simulink model "EngTemplate_r2017a"  (R2017a)
settings: Solver=ode5  StartTime=0.0  StopTime=inf  FixedStep=0.0001  RelTol=1e-3  EnableMultiTasking=on
values from neighbouring files (symbols this model uses):
  Patm = 101.3e3    (= 101300)    [EngineParameters.m]
settings Model: Creator=bamason2  LastModifiedBy=byronmason
settings DataIOCC: LimitDataPoints=on  SaveFormat=Array
settings OptimizationCC: LifeSpan=inf
settings DebuggingCC: SFUnexpectedBacktrackingDiag=warning  SFNoUnconditionalDefaultTransitionDiag=warning  SFExecutionAtInitializationDiag=none
settings HardwareCC: ProdBitPerPointer=32  ProdBitPerSizeT=32  ProdBitPerPtrDiffT=32  ProdLargestAtomicFloat=None  ProdIntDivRoundTo=Undefined  ProdEndianess=Unspecified  ProdWordSize=32  ProdHWDeviceType=32-bit Generic
settings ModelReferenceCC: PropagateSignalLabelsOutOfModel=off
settings GRTTargetCC: TargetLangStandard=C89/C90 (ANSI)
settings ConfigComp: CovMetricSettings=dw  CovSaveCumulativeToWorkspaceVar=on  CovSaveSingleToWorkspaceVar=on  CovExternalEMLEnable=off

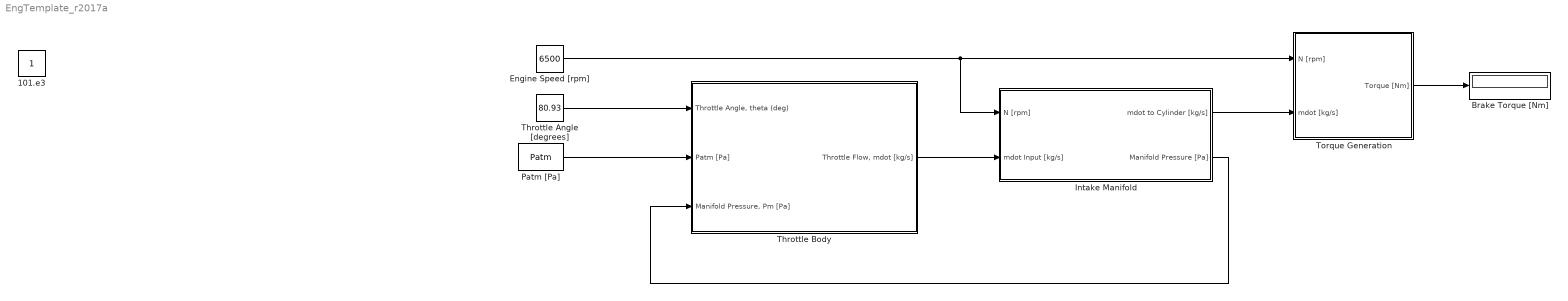
== system EngTemplate_r2017a ==
  Brake Torque [Nm] : Display
  Engine Speed [rpm] : Constant  Value=6500
  Intake Manifold : Subsystem
  Patm [Pa] : Constant  Value=Patm
  Throttle Angle [degrees] : Constant  Value=80.93
  Throttle Body : Subsystem
  Torque Generation : Subsystem
  101.e3 : Constant  IOType=siggen
  wires:
  Intake Manifold/1(mdot to Cylinder [kg/s]) -> Torque Generation/2(mdot [kg/s])
  Torque Generation/1(Torque [Nm]) -> Brake Torque [Nm]/1
  Intake Manifold/2(Manifold Pressure [Pa]) -> Throttle Body/3("Manifold Pressure, Pm [Pa]")
  Throttle Body/1("Throttle Flow, mdot [kg/s]") -> Intake Manifold/2(mdot Input [kg/s])
  Engine Speed [rpm]/1 -> Intake Manifold/1(N [rpm]), Torque Generation/1(N [rpm])
  Throttle Angle [degrees]/1 -> Throttle Body/1("Throttle Angle, theta (deg)")
  Patm [Pa]/1 -> Throttle Body/2(Patm [Pa])

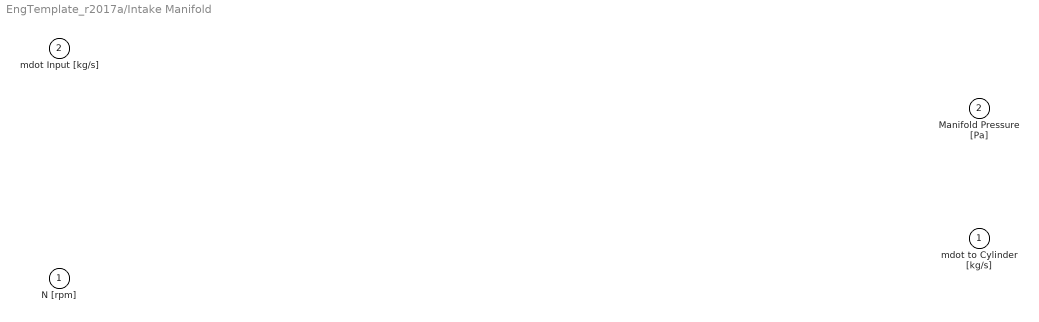
== system EngTemplate_r2017a/Intake Manifold ==
  N [rpm] : Inport
  mdot Input [kg/s] : Inport  Port=2
  mdot to Cylinder [kg/s] : Outport  InitialOutput=0
  Manifold Pressure [Pa] : Outport  Port=2  InitialOutput=0

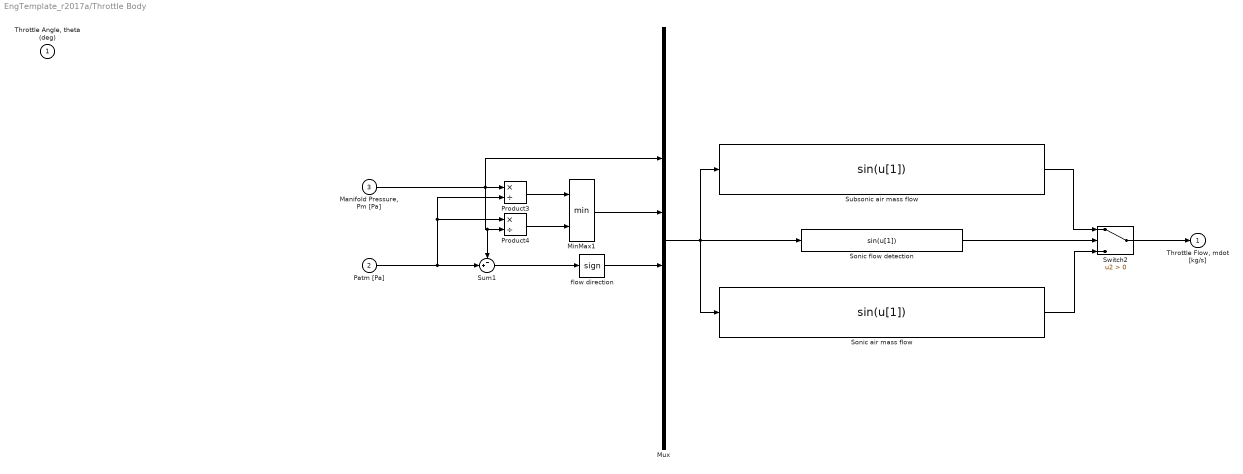
== system EngTemplate_r2017a/Throttle Body ==
  "Throttle Angle, theta (deg)" : Inport
  Patm [Pa] : Inport  Port=2
  "Manifold Pressure, Pm [Pa]" : Inport  Port=3
  MinMax1 : MinMax  Inputs=2  InputSameDT=on  SaturateOnIntegerOverflow=on
  Mux : Mux  Inputs=8
  Product3 : Product  Inputs=*/  InputSameDT=on  RndMeth=Zero  SaturateOnIntegerOverflow=on  OutDataTypeStr=Inherit: Same as first input
  Product4 : Product  Inputs=*/  InputSameDT=on  RndMeth=Zero  SaturateOnIntegerOverflow=on  OutDataTypeStr=Inherit: Same as first input
  Sonic air mass flow : Fcn
  Sonic flow detection : Fcn
  Subsonic air mass flow : Fcn
  Sum1 : Sum  Inputs=-+|  InputSameDT=on  SaturateOnIntegerOverflow=on  OutDataTypeStr=Inherit: Same as first input
  Switch2 : Switch  Criteria=u2 > Threshold
  flow direction : Signum
  "Throttle Flow, mdot [kg/s]" : Outport  InitialOutput=0
  wires:
  Mux/1 -> Sonic air mass flow/1, Subsonic air mass flow/1, Sonic flow detection/1
  Sonic flow detection/1 -> Switch2/2
  Switch2/1 -> "Throttle Flow, mdot [kg/s]"/1
  Subsonic air mass flow/1 -> Switch2/1
  Sonic air mass flow/1 -> Switch2/3
  "Manifold Pressure, Pm [Pa]"/1 -> Product4/2, Sum1/1, Mux/3, Product3/1
  flow direction/1 -> Mux/5
  Patm [Pa]/1 -> Product4/1, Product3/2, Sum1/2
  Sum1/1 -> flow direction/1
  Product4/1 -> MinMax1/2
  MinMax1/1 -> Mux/4
  Product3/1 -> MinMax1/1

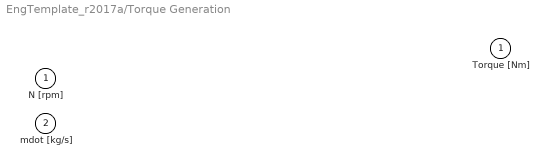
== system EngTemplate_r2017a/Torque Generation ==
  N [rpm] : Inport
  mdot [kg/s] : Inport  Port=2
  Torque [Nm] : Outport  InitialOutput=0
